simulink model "DRScreeningFlow"  (R2026a)
settings: Solver=VariableStepAuto  StopTime=480
undefined symbols (not defined in the file or in its folder): exprnd, m, n
settings Model: Creator=ruhan  LastModifiedBy=ruhan

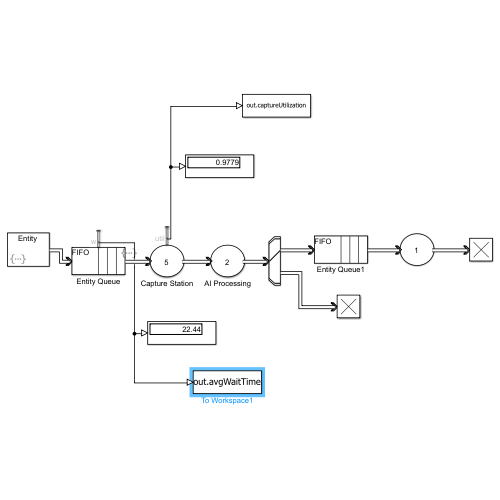
[thumbnail: Simulink's stored preview of the top-level diagram]
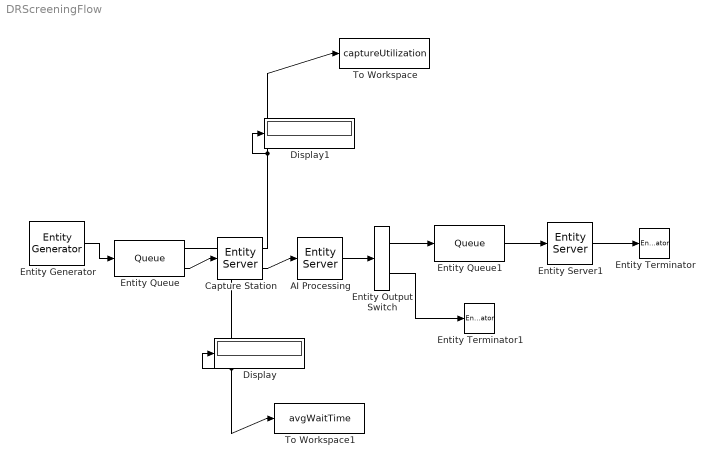
== system DRScreeningFlow ==
  AI Processing : EntityServer  InputPortMessageModes=m  OutputPortMessageModes=m  Capacity=2  ServiceTimeValue=exprnd(2.5)
  Capture Station : EntityServer  InputPortMessageModes=m  OutputPortMessageModes=n,m  ServiceTimeValue=exprnd(5)  EntryAction=|  Utilization=on
      | if rand < 0.20
      |     entity.RoutingPort = 1;
      | else
      |     entity.RoutingPort = 2;
      | end
      settings: OutputPortMap=o5,o9
  Display : Display
  Display1 : Display
  Entity Output Switch : EntityOutputSwitch  InputPortMessageModes=m  OutputPortMessageModes=m,m  SwitchingCriterion=From attribute  SwitchAttributeName=RoutingPort
  Entity Generator : EntityGenerator  OutputPortMessageModes=m  Period=1.2  GenerateAction=entity.RoutingPort = 1;  AttributeName=Attribute1|RoutingPort  AttributeInitialValue=1|1  EntityType=Structured  EntityTypeName=Entity
  Entity Queue : Queue  InputPortMessageModes=m  OutputPortMessageModes=n,m  Capacity=inf  AverageWait=on
      settings: OutputPortMap=o2,o5
  Entity Queue1 : Queue  InputPortMessageModes=m  OutputPortMessageModes=m
  Entity Server1 : EntityServer  InputPortMessageModes=m  OutputPortMessageModes=m  Capacity=1  ServiceTimeValue=exprnd(0.5)
  Entity Terminator : EntityTerminator  InputPortMessageModes=m
  Entity Terminator1 : EntityTerminator  InputPortMessageModes=m
  To Workspace : ToWorkspace  VariableName=captureUtilization  SampleTime=-1
  To Workspace1 : ToWorkspace  VariableName=avgWaitTime  SampleTime=-1
  wires:
  Entity Generator/1 -> Entity Queue/1
  Entity Queue/2 -> Capture Station/1
  Capture Station/2 -> AI Processing/1
  Entity Queue/1 -> To Workspace1/1, Display/1
  Capture Station/1 -> To Workspace/1, Display1/1
  Entity Output Switch/1 -> Entity Queue1/1
  Entity Queue1/1 -> Entity Server1/1
  Entity Output Switch/2 -> Entity Terminator1/1
  Entity Server1/1 -> Entity Terminator/1
  AI Processing/1 -> Entity Output Switch/1
